simulink model "TL1_cs"  (R2019a)
settings: Solver=FixedStepDiscrete  StartTime=0.0  StopTime=40  FixedStep=1/300  RelTol=1e-3
PreLoadFcn:
  | mbxruntime.callbacks.PreLoadFcn(bdroot);
  | check_NUTS_defined
  | model_closed = 0;
  | assignin('base',['model_closed_' bdroot],false);
PostLoadFcn:
  | mbxruntime.callbacks.PostLoadFcn(bdroot);
InitFcn:
  | mbxruntime.callbacks.InitFcn(bdroot);
StartFcn:
  | mbxruntime.callbacks.StartFcn(bdroot);
StopFcn:
  | mbxruntime.callbacks.StopFcn(bdroot);;
  | 
model workspace: external: MAT-File .\TL1_cs_hws.mat (data not in the file)
undefined symbols (not defined in the file): AngularVelocity, Clock_, Data, Data_SL_Info, DiscIntNeverNeededParam, Encoding, Encoding_SL_Info, Header, Height, InitImageOutputDir, LinearAcceleration, mbxruntime, Orientation, Pose, Poses, Poses_SL_Info, Position, Step, tabledata, Twist, Width
libraries: robotlib x24, simulink_extras x16, PreScanSimulinkLibrary x4, dspindex x4, robotcorelib x2, visionconversions x2, visionsinks x2, sharedtransform x1
(part 2 of 4)

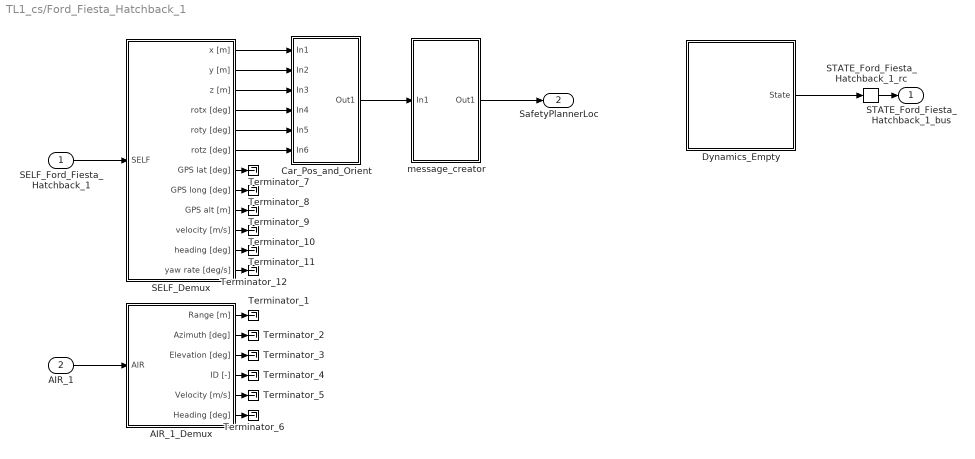
== system TL1_cs/Ford_Fiesta_Hatchback_1 ==
  SELF_Ford_Fiesta_Hatchback_1 : Inport  Tag=inport/SelfPort  OutDataTypeStr=Bus: PRESCAN_SELFSENSORDATA  PortDimensions=1  SampleTime=1/300  BusOutputAsStruct=on
  AIR_1 : Inport  Tag=inport/AIR  Port=2  OutDataTypeStr=Bus: PRESCAN_AIRSENSORMESSAGE  PortDimensions=1  SampleTime=1/300  BusOutputAsStruct=on
  AIR_1_Demux : Subsystem  Tag=demux/AIR  mask(PreScan Demux Block: AIR){DetectionType=BBox, detectableObjects=1}
      mask prompts: DetectionType "Detection Type"; detectableObjects "Max. detectable objects"
      mask help:
      | The Actor Information Receiver sensor provides a fast, simple and generic detection solution which is not tied up to a specific technology and can be used for scenarios in which a simple sensor is needed.
      |
      | For more information, please click Help.
      mask init:
      | switch DetectionType
      |     case 1
      |         DetectionTypeStr = 'Center';
      |     case 2
      |         DetectionTypeStr = 'BBox';
      |     case 3
      |         DetectionTypeStr = 'CoG';
      |     otherwise
      |         DetectionTypeStr = 'Unknown';
      | end
      settings: DeleteFcn=PreScanBlockDeleteFcn;
      mask Help: eval('openHelp(413)')
      mask TypeOptions DetectionType: Center | BBox | CoG
      mask Display:
      | disp(char('Det. type:         ',['{\it',DetectionTypeStr,'}']),'texmode','on')
      | port_label('output',1,'Range [m]')
      | port_label('output',2,'{\theta} [deg]','texmode','on')
      | port_label('output',3,'{\phi} [deg]','texmode','on')
      | port_label('output',4,'ID [-]','texmode','on')
      | port_label('output',5,'Velocity [m/s]','texmode','on')
      | port_label('output',6,'Heading [deg]','texmode','on')
  Car_Pos_and_Orient : Subsystem
  Dynamics_Empty : Subsystem  Tag=Dynamics_Empty
      mask Help: eval('openHelp(202)')
      mask Display: port_label('output', 1, 'State');text(0,0,' Empty\n')
  SELF_Demux : Subsystem  Tag=demux/SelfPort  mask(PreScan Demux Block:){}
      mask help:
      | The SELF port shows (state) information of the actor itself. The outputs are position in the experiment's axis system and the GPS coordinates, and the object's absolute velocity and compass heading.
      |
      | For more information, please click Help.
      settings: DeleteFcn=PreScanBlockDeleteFcn;
      mask Help: eval('openHelp(462)')
      mask Display:
      | port_label('output',1,'x [m]')
      | port_label('output',2,'y [m]')
      | port_label('output',3,'z [m]','texmode','on')
      | port_label('output',4,'Rotx [deg]','texmode','on')
      | port_label('output',5,'Roty [deg]','texmode','on')
      | port_label('output',6,'Rotz [deg]','texmode','on')
      | port_label('output',7,'GPS lat [deg]','texmode','on')
      | port_label('output',8,'GPS long [deg]','texmode','on')
      | port_label('output',9,'GPS alt [m]','texmode','on')
      | port_label('output',10,'Velocity [m/s]')
      | port_label('output',11,'Heading [deg]')
      | port_label('output',12,'Yaw rate [deg/s]')
  STATE_Ford_Fiesta_Hatchback_1_rc : RateTransition  Tag=mux_rc/StatePort  OutPortSampleTimeOpt=Inherit
  Terminator_{1..12} (12 alike) : Terminator
  message_creator : Subsystem
  STATE_Ford_Fiesta_Hatchback_1_bus : Outport  Tag=outport/StatePort  OutDataTypeStr=Bus: PRESCAN_STATEACTUATORDATA  PortDimensions=1  SampleTime=1/300
  SafetyPlannerLoc : Outport  Port=2
  wires:
  Car_Pos_and_Orient/1(Out1) -> message_creator/1(In1)
  message_creator/1(Out1) -> SafetyPlannerLoc/1
  SELF_Demux/1(x [m]) -> Car_Pos_and_Orient/1(In1)
  SELF_Demux/2(y [m]) -> Car_Pos_and_Orient/2(In2)
  SELF_Demux/3(z [m]) -> Car_Pos_and_Orient/3(In3)
  SELF_Demux/4(rotx [deg]) -> Car_Pos_and_Orient/4(In4)
  SELF_Demux/5(roty [deg]) -> Car_Pos_and_Orient/5(In5)
  SELF_Demux/6(rotz [deg]) -> Car_Pos_and_Orient/6(In6)
  STATE_Ford_Fiesta_Hatchback_1_rc/1 -> STATE_Ford_Fiesta_Hatchback_1_bus/1
  SELF_Ford_Fiesta_Hatchback_1/1 -> SELF_Demux/1(SELF)
  AIR_1/1 -> AIR_1_Demux/1(AIR)
  Dynamics_Empty/1(State) -> STATE_Ford_Fiesta_Hatchback_1_rc/1
  AIR_1_Demux/1(Range [m]) -> Terminator_1/1
  AIR_1_Demux/2(Azimuth [deg]) -> Terminator_2/1
  AIR_1_Demux/3(Elevation [deg]) -> Terminator_3/1
  AIR_1_Demux/4(ID [-]) -> Terminator_4/1
  AIR_1_Demux/5(Velocity [m/s]) -> Terminator_5/1
  AIR_1_Demux/6(Heading [deg]) -> Terminator_6/1
  SELF_Demux/7(GPS lat [deg]) -> Terminator_7/1
  SELF_Demux/8(GPS long [deg]) -> Terminator_8/1
  SELF_Demux/9(GPS alt [m]) -> Terminator_9/1
  SELF_Demux/10(velocity [m/s]) -> Terminator_10/1
  SELF_Demux/11(heading [deg]) -> Terminator_11/1
  SELF_Demux/12(yaw rate [deg/s]) -> Terminator_12/1

== system TL1_cs/HumViewCamera ==
  Sensor : S-Function  FunctionName=sfun_Camera  Parameters=sensorID, dataWidth, dataHeight, channelsPerImage, numberOfImages, timestep  SFunctionDeploymentMode=off  EnableBusSupport=off  mask(PreScan Source Block: Camera Sensor){sensorID=14458, dataWidth=1080, dataHeight=5613, channelsPerImage=3, numberOfImages=1, timestep=1/60}
      mask prompts: sensorID "Sensor ID"; dataWidth "Data width"; dataHeight "Data Height"; channelsPerImage "Channels per image"; numberOfImages "Number of images"; timestep "MATLAB timestep:"
      mask help: The Camera Sensor provides a color or monochrome image.
      mask Help: eval('openHelp(457)')
      mask Display: image(imread('CameraSensor.png'))
  HumViewCamera : Outport  Tag=outport/Camera/CameraSensor  OutDataTypeStr=uint8  SampleTime=1/60
  wires:
  Sensor/1 -> HumViewCamera/1

== system TL1_cs/PointCloudSensor_1 ==
  Sensor : S-Function  FunctionName=sfun_PCS  Parameters=sensorID, dataWidth, dataHeight, numChannels, dataType, timestep  SFunctionDeploymentMode=off  EnableBusSupport=off  mask(PreScan Source Block: Point Cloud Sensor){sensorID=9052, dataWidth=16, dataHeight=900, numChannels=4, dataType=0, timestep=1/20}
      mask prompts: sensorID "Sensor ID"; dataWidth "Data Width"; dataHeight "Data Height"; numChannels "Channel Count"; dataType "Data Type"; timestep "MATLAB timestep:"
      mask help: The Point Cloud Sensor provides XYZ positions relative to the sensor
      mask Help: eval('openHelp(6400)')
      mask Display: image(imread('PointCloudSensorSL.png'))
  PointCloudSensor_1 : Outport  Tag=outport/PointCloudInport  OutDataTypeStr=single  SampleTime=1/20
  wires:
  Sensor/1 -> PointCloudSensor_1/1

== system TL1_cs/PointCloudSensor_2 ==
  Sensor : S-Function  FunctionName=sfun_PCS  Parameters=sensorID, dataWidth, dataHeight, numChannels, dataType, timestep  SFunctionDeploymentMode=off  EnableBusSupport=off  mask(PreScan Source Block: Point Cloud Sensor){sensorID=9053, dataWidth=16, dataHeight=900, numChannels=4, dataType=0, timestep=1/20}
      mask prompts: sensorID "Sensor ID"; dataWidth "Data Width"; dataHeight "Data Height"; numChannels "Channel Count"; dataType "Data Type"; timestep "MATLAB timestep:"
      mask help: The Point Cloud Sensor provides XYZ positions relative to the sensor
      mask Help: eval('openHelp(6400)')
      mask Display: image(imread('PointCloudSensorSL.png'))
  PointCloudSensor_2 : Outport  Tag=outport/PointCloudInport  OutDataTypeStr=single  SampleTime=1/20
  wires:
  Sensor/1 -> PointCloudSensor_2/1

== system TL1_cs/PointCloudSensor_3 ==
  Sensor : S-Function  FunctionName=sfun_PCS  Parameters=sensorID, dataWidth, dataHeight, numChannels, dataType, timestep  SFunctionDeploymentMode=off  EnableBusSupport=off  mask(PreScan Source Block: Point Cloud Sensor){sensorID=9054, dataWidth=16, dataHeight=900, numChannels=4, dataType=0, timestep=1/20}
      mask prompts: sensorID "Sensor ID"; dataWidth "Data Width"; dataHeight "Data Height"; numChannels "Channel Count"; dataType "Data Type"; timestep "MATLAB timestep:"
      mask help: The Point Cloud Sensor provides XYZ positions relative to the sensor
      mask Help: eval('openHelp(6400)')
      mask Display: image(imread('PointCloudSensorSL.png'))
  PointCloudSensor_3 : Outport  Tag=outport/PointCloudInport  OutDataTypeStr=single  SampleTime=1/20
  wires:
  Sensor/1 -> PointCloudSensor_3/1

== system TL1_cs/PointCloudSensor_4 ==
  Sensor : S-Function  FunctionName=sfun_PCS  Parameters=sensorID, dataWidth, dataHeight, numChannels, dataType, timestep  SFunctionDeploymentMode=off  EnableBusSupport=off  mask(PreScan Source Block: Point Cloud Sensor){sensorID=9055, dataWidth=16, dataHeight=900, numChannels=4, dataType=0, timestep=1/20}
      mask prompts: sensorID "Sensor ID"; dataWidth "Data Width"; dataHeight "Data Height"; numChannels "Channel Count"; dataType "Data Type"; timestep "MATLAB timestep:"
      mask help: The Point Cloud Sensor provides XYZ positions relative to the sensor
      mask Help: eval('openHelp(6400)')
      mask Display: image(imread('PointCloudSensorSL.png'))
  PointCloudSensor_4 : Outport  Tag=outport/PointCloudInport  OutDataTypeStr=single  SampleTime=1/20
  wires:
  Sensor/1 -> PointCloudSensor_4/1

== system TL1_cs/PreScanTerminator ==
  Terminator : Terminator
  sfun_Terminator : S-Function  FunctionName=sfun_Terminator  Parameters=SampleTime  SFunctionDeploymentMode=off  EnableBusSupport=off  mask(Legacy Function){SFunctionSpec=void prescan_terminator_outputFcn(void ** work1, PRESCAN_TERMINATORDATA y1[1]), SampleTime=TimeStep, ShowSpec=on}
      mask prompts: SampleTime "Sample time (-1 for inherited):"; ShowSpec "Display function specification"
      mask help:
      | This block allows you to call the legacy functions specified by the following Legacy Code Tool definition:
      | def.SFunctionName = 'sfun_Terminator';
      | def.OutputFcnSpec = 'void prescan_terminator_outputFcn(void ** work1, PRESCAN_TERMINATORDATA y1[1])';
      | def.StartFcnSpec = 'void prescan_terminator_startFcn(void ** work1)';
      | def.TerminateFcnSpec = 'void prescan_terminator_terminateFcn(void ** work1)';
      | def.HeaderFiles = {'prescan_terminator_data.h'};
      | def.HostLibFiles = {'sensorinterfaced.lib'};
      | def.IncPaths = {'src', 'C:\prescandev\vislibrary\vis\..\pimp\include\sensors\InterfaceRTW'};
      | def.SrcPaths = {'src'};
      | def.LibPaths = {'C:\\prescandev\\vislibrary_build\lib'};
      | def.SampleTime = 'parameterized';
      | def.Options.language = 'C';
      mask Help: <p>This block was generated automatically by the Legacy Code Tool. For detailed help on this tool, call<a href="matlab:legacy_code('help')"> legacy_code('help')</a>.</p>
      mask Callback ShowSpec:
      | if strcmp(get_param(gcbh, 'ShowSpec'), 'on')
      |   set_param(gcbh, 'MaskDisplay', sprintf('fprintf(''%s'');', get_param(gcbh, 'SFunctionSpec')));
      | else
      |   set_param(gcbh, 'MaskDisplay', sprintf('fprintf(''%s'');', get_param(gcbh, 'FunctionName')));
      | end
      mask Display: fprintf('void prescan_terminator_outputFcn(void ** work1, PRESCAN_TERMINATORDATA y1[1])');
  wires:
  sfun_Terminator/1 -> Terminator/1

== system TL1_cs/SELF_BMW_X5_SUV_1 ==
  Sensor : S-Function  FunctionName=sfun_SelfSensor  Parameters=UniqueID, TimeStep  SFunctionDeploymentMode=off  EnableBusSupport=off  mask(PreScan Source Block: SELF){UniqueID=9040, TimeStep=1/300}
      mask prompts: UniqueID "Auto-Assigned: Unique ID"; TimeStep "Auto-Assigned: Upload Period [s]"
      mask help:
      | The SELF port shows (state) information of the actor itself. The outputs are position in the experiment's axis system and the GPS coordinates, and the object's absolute velocity and compass heading.
      |
      | For more information, please click Help.
      mask Help: eval('openHelp(462)')
      mask Display: image(imread('GPS.png'))
  SELF_BMW_X5_SUV_1 : Outport  Tag=outport/SelfPort  OutDataTypeStr=Bus: PRESCAN_SELFSENSORDATA  PortDimensions=1  SampleTime=1/300
  wires:
  Sensor/1 -> SELF_BMW_X5_SUV_1/1

== system TL1_cs/SELF_Ford_Fiesta_Hatchback_1 ==
  Sensor : S-Function  FunctionName=sfun_SelfSensor  Parameters=UniqueID, TimeStep  SFunctionDeploymentMode=off  EnableBusSupport=off  mask(PreScan Source Block: SELF){UniqueID=4876, TimeStep=1/300}
      mask prompts: UniqueID "Auto-Assigned: Unique ID"; TimeStep "Auto-Assigned: Upload Period [s]"
      mask help:
      | The SELF port shows (state) information of the actor itself. The outputs are position in the experiment's axis system and the GPS coordinates, and the object's absolute velocity and compass heading.
      |
      | For more information, please click Help.
      mask Help: eval('openHelp(462)')
      mask Display: image(imread('GPS.png'))
  SELF_Ford_Fiesta_Hatchback_1 : Outport  Tag=outport/SelfPort  OutDataTypeStr=Bus: PRESCAN_SELFSENSORDATA  PortDimensions=1  SampleTime=1/300
  wires:
  Sensor/1 -> SELF_Ford_Fiesta_Hatchback_1/1

== system TL1_cs/STATE_BMW_X5_SUV_1_bus ==
  STATE_BMW_X5_SUV_1_bus : Inport  Tag=inport/StatePort  OutDataTypeStr=Bus: PRESCAN_STATEACTUATORDATA  PortDimensions=1  SampleTime=1/300  BusOutputAsStruct=on
  Actuator : S-Function  FunctionName=sfun_StateActuator  Parameters=UniqueID, TimeStep  SFunctionDeploymentMode=off  EnableBusSupport=off  mask(PreScan Sink Block: State){UniqueID=9040, TimeStep=1/300}
      mask prompts: UniqueID "Auto-Assigned: Unique ID"; TimeStep "Auto-Assigned: Upload Period [s]"
      mask help:
      | The Actor State contains a vector signal of size (9x1), containing the following signals:
      |
      | -  Position    	(x,y,z)             	[m]
      | -  Velocity    	(vx,vy,vz)         	[m/s]
      | -  Angles       	(Roll, Pitch, Yaw)	[rad]
      |
      | The Actor state is defined in the global axis system.
      | The state is superponed on the Initial position defined in the GUI.
      |
      | For more information, please click Help.
      mask Help: eval('openHelp(222)')
      mask Display: image(imread('State.png'))
  wires:
  STATE_BMW_X5_SUV_1_bus/1 -> Actuator/1

== system TL1_cs/STATE_Ford_Fiesta_Hatchback_1_bus ==
  STATE_Ford_Fiesta_Hatchback_1_bus : Inport  Tag=inport/StatePort  OutDataTypeStr=Bus: PRESCAN_STATEACTUATORDATA  PortDimensions=1  SampleTime=1/300  BusOutputAsStruct=on
  Actuator : S-Function  FunctionName=sfun_StateActuator  Parameters=UniqueID, TimeStep  SFunctionDeploymentMode=off  EnableBusSupport=off  mask(PreScan Sink Block: State){UniqueID=4876, TimeStep=1/300}
      mask prompts: UniqueID "Auto-Assigned: Unique ID"; TimeStep "Auto-Assigned: Upload Period [s]"
      mask help:
      | The Actor State contains a vector signal of size (9x1), containing the following signals:
      |
      | -  Position    	(x,y,z)             	[m]
      | -  Velocity    	(vx,vy,vz)         	[m/s]
      | -  Angles       	(Roll, Pitch, Yaw)	[rad]
      |
      | The Actor state is defined in the global axis system.
      | The state is superponed on the Initial position defined in the GUI.
      |
      | For more information, please click Help.
      mask Help: eval('openHelp(222)')
      mask Display: image(imread('State.png'))
  wires:
  STATE_Ford_Fiesta_Hatchback_1_bus/1 -> Actuator/1

== system TL1_cs/Synchronizer ==
  Bus Selector1 : BusSelector  OutputSignals=FederateStopped
  Stop Simulation : Stop
  sfun_Synchronizer : S-Function  FunctionName=sfun_Synchronizer  Parameters=SampleTime  SFunctionDeploymentMode=off  EnableBusSupport=off  mask(Legacy Function){SFunctionSpec=void prescan_synchronizer_outputFcn(void ** work1, PRESCAN_SYNCHRONIZEDATA y1[1]), SampleTime=TimeStep, ShowSpec=on}
      mask prompts: SampleTime "Sample time (-1 for inherited):"; ShowSpec "Display function specification"
      mask help:
      | This block allows you to call the legacy functions specified by the following Legacy Code Tool definition:
      | def.SFunctionName = 'sfun_Synchronizer';
      | def.OutputFcnSpec = 'void prescan_synchronizer_outputFcn(void ** work1, PRESCAN_SYNCHRONIZEDATA y1[1])';
      | def.StartFcnSpec = 'void prescan_synchronizer_startFcn(void ** work1)';
      | def.TerminateFcnSpec = 'void prescan_synchronizer_terminateFcn(void ** work1)';
      | def.HeaderFiles = {'prescan_synchronizer_data.h'};
      | def.HostLibFiles = {'sensorinterfaced.lib'};
      | def.IncPaths = {'src', 'C:\prescandev\vislibrary\vis\..\pimp\include\sensors\InterfaceRTW'};
      | def.SrcPaths = {'src'};
      | def.LibPaths = {'C:\\prescandev\\vislibrary_build\lib'};
      | def.SampleTime = 'parameterized';
      | def.Options.language = 'C';
      mask Help: <p>This block was generated automatically by the Legacy Code Tool. For detailed help on this tool, call<a href="matlab:legacy_code('help')"> legacy_code('help')</a>.</p>
      mask Callback ShowSpec:
      | if strcmp(get_param(gcbh, 'ShowSpec'), 'on')
      |   set_param(gcbh, 'MaskDisplay', sprintf('fprintf(''%s'');', get_param(gcbh, 'SFunctionSpec')));
      | else
      |   set_param(gcbh, 'MaskDisplay', sprintf('fprintf(''%s'');', get_param(gcbh, 'FunctionName')));
      | end
      mask Display: fprintf('void prescan_synchronizer_outputFcn(void ** work1, PRESCAN_SYNCHRONIZEDATA y1[1])');
  wires:
  Bus Selector1/1 -> Stop Simulation/1  "<FederateStopped>"
  sfun_Synchronizer/1 -> Bus Selector1/1

== system TL1_cs/TrafficLightRoadSideNL_1 ==
  Constant : Constant
  Ground_1 : Ground
  Ground_2 : Ground
  VISUCasingLights_Mux : Subsystem  Tag=mux/VisuCasingLights  mask(PreScan User Interface: VisuTrafficLight){}
      mask help:
      | The VisuTrafficLight block provides a way to animate traffic lights: switch on and off individual lights.
      |
      | For more information, please click Help.
      mask Help: eval('openHelp(731)')
  VISUCasingLights_TrafficLightRoadSideNL_1 : Outport  Tag=outport/VisuCasingLights  SampleTime=1/300
  wires:
  VISUCasingLights_Mux/1(VISUCasingLights_TrafficLightRoadSideNL_1) -> VISUCasingLights_TrafficLightRoadSideNL_1/1
  Ground_1/1 -> VISUCasingLights_Mux/1(Green [-])
  Ground_2/1 -> VISUCasingLights_Mux/2(Orange [-])
  Constant/1 -> VISUCasingLights_Mux/3(Red [-])

== system TL1_cs/VISUCasingLights_TrafficLightRoadSideNL_1 ==
  VISUCasingLights_TrafficLightRoadSideNL_1 : Inport  Tag=inport/VisuCasingLights  SampleTime=1/300  BusOutputAsStruct=on
  Actuator : Subsystem  mask(PreScan Sink Block: VisuTrafficLight){UniqueID=20538, ColorsObjectQuery=, Colors=[]}
      mask prompts: UniqueID "Parent Unique Identifier"; ColorsObjectQuery "Query for Color Object"; Colors "Matrix of colors"
      mask help:
      | The VisuTrafficLight block provides a way to animate traffic lights: switch on and off individual lights.
      |
      | For more information, please click Help.
      mask Help: eval('openHelp(731)')
      mask Display: image(imread('TrafficLightCasing.png'))
  wires:
  VISUCasingLights_TrafficLightRoadSideNL_1/1 -> Actuator/1(VISUCasingLights_TrafficLightRoadSideNL_1)

== system TL1_cs/camera ==
  Sensor : S-Function  FunctionName=sfun_Camera  Parameters=sensorID, dataWidth, dataHeight, channelsPerImage, numberOfImages, timestep  SFunctionDeploymentMode=off  EnableBusSupport=off  mask(PreScan Source Block: Camera Sensor){sensorID=9056, dataWidth=720, dataHeight=2880, channelsPerImage=3, numberOfImages=1, timestep=1/20}
      mask prompts: sensorID "Sensor ID"; dataWidth "Data width"; dataHeight "Data Height"; channelsPerImage "Channels per image"; numberOfImages "Number of images"; timestep "MATLAB timestep:"
      mask help: The Camera Sensor provides a color or monochrome image.
      mask Help: eval('openHelp(457)')
      mask Display: image(imread('CameraSensor.png'))
  camera : Outport  Tag=outport/Camera/CameraSensor  OutDataTypeStr=uint8  SampleTime=1/20
  wires:
  Sensor/1 -> camera/1

== system TL1_cs/pose_otheCar ==
  In1 : Inport
  Enable : EnablePort
  Add5 : Sum
  Assignment : Assignment  OutputInitialize=Specify size for each dimension in table  DiagnosticForDimensions=Warning  IndexOptions=Starting index (dialog)  Indices=1  OutputSizes=1
  Assignment2 : Assignment  OutputInitialize=Specify size for each dimension in table  DiagnosticForDimensions=Warning  IndexOptions=Starting index (dialog)  Indices=1  OutputSizes=1000
  Blank Message1 : robotlib/Blank Message  messageClass=Message  entityType=geometry_msgs/PoseArray  messageType=geometry_msgs/PoseArray  SampleTime=inf
      settings: SourceProductBaseCode=RO
  Bus Assignment3 : BusAssignment  AssignedSignals=Header.Seq,Header.FrameId,Header.FrameId_SL_Info.CurrentLength,Poses,Poses_SL_Info.CurrentLength
  Bus Selector : BusSelector  OutputSignals=Poses
  Bus Selector2 : BusSelector  OutputSignals=Header.FrameId
  Constant24 : Constant  OutDataTypeStr=uint32
  Constant25 : Constant  Value=uint8(['map'])
  Memory2 : Memory  InheritSampleTime=on
  Publish2 : robotlib/Publish  topicSource=Specify your own  topic=/pose_otherCar  messageType=geometry_msgs/PoseArray  messageQueueLength=1
      settings: SourceProductBaseCode=RO
  Width : Width  DataType=uint32
  Width5 : Width  DataType=uint32
  wires:
  Constant24/1 -> Add5/2
  Memory2/1 -> Add5/1
  Add5/1 -> Bus Assignment3/2, Memory2/1
  Width5/1 -> Bus Assignment3/4
  Assignment/1 -> Bus Assignment3/5, Width/1
  Width/1 -> Bus Assignment3/6
  Bus Selector/1 -> Assignment/1  "<Poses>"
  In1/1 -> Assignment/2
  Bus Assignment3/1 -> Publish2/1
  Constant25/1 -> Assignment2/2
  Assignment2/1 -> Bus Assignment3/3, Width5/1
  Bus Selector2/1 -> Assignment2/1  "<FrameId>"
  Blank Message1/1 -> Bus Selector/1, Bus Selector2/1, Bus Assignment3/1

== system TL1_cs/tl_camera ==
  Sensor : S-Function  FunctionName=sfun_Camera  Parameters=sensorID, dataWidth, dataHeight, channelsPerImage, numberOfImages, timestep  SFunctionDeploymentMode=off  EnableBusSupport=off  mask(PreScan Source Block: Camera Sensor){sensorID=12017, dataWidth=720, dataHeight=2880, channelsPerImage=3, numberOfImages=1, timestep=1/20}
      mask prompts: sensorID "Sensor ID"; dataWidth "Data width"; dataHeight "Data Height"; channelsPerImage "Channels per image"; numberOfImages "Number of images"; timestep "MATLAB timestep:"
      mask help: The Camera Sensor provides a color or monochrome image.
      mask Help: eval('openHelp(457)')
      mask Display: image(imread('CameraSensor.png'))
  tl_camera : Outport  Tag=outport/Camera/CameraSensor  OutDataTypeStr=uint8  SampleTime=1/20
  wires:
  Sensor/1 -> tl_camera/1

== system TL1_cs/BMW_X5_SUV_1/Car_Pose ==
  In1 : Inport
  In2 : Inport  Port=2
  In3 : Inport  Port=3
  In4 : Inport  Port=4
  In5 : Inport  Port=5
  In6 : Inport  Port=6
  Coordinate Transformation Conversion : robotcorelib/Coordinate Transformation Conversion  InputRepresentation=Euler Angles  InputEulerSequence=XYZ  ShowTrVecInputPort=on  OutputRepresentation=Quaternion  OutputEulerSequence=ZYX  ShowTrVecOutputPort=on  SimulateUsing=Interpreted execution
      settings: SourceProductBaseCode=RO
  Data Type Conversion : DataTypeConversion
  Data Type Conversion1 : DataTypeConversion
  Data Type Conversion2 : DataTypeConversion
  Degrees to Radians1 : simulink_extras/Transformations/Degrees to Radians
  Degrees to Radians2 : simulink_extras/Transformations/Degrees to Radians
  Degrees to Radians5 : simulink_extras/Transformations/Degrees to Radians
  Mux : Mux
  Vector Concatenate2 : Concatenate  NumInputs=3
  Out1 : Outport
  wires:
  Mux/1 -> Out1/1
  Coordinate Transformation Conversion/1 -> Mux/4
  Data Type Conversion2/1 -> Mux/3
  Data Type Conversion1/1 -> Mux/2
  Data Type Conversion/1 -> Mux/1
  In6/1 -> Degrees to Radians2/1
  In5/1 -> Degrees to Radians1/1
  In4/1 -> Degrees to Radians5/1
  In3/1 -> Data Type Conversion2/1
  In2/1 -> Data Type Conversion1/1
  In1/1 -> Data Type Conversion/1
  Degrees to Radians2/1 -> Vector Concatenate2/3
  Vector Concatenate2/1 -> Coordinate Transformation Conversion/1
  Degrees to Radians5/1 -> Vector Concatenate2/1
  Degrees to Radians1/1 -> Vector Concatenate2/2

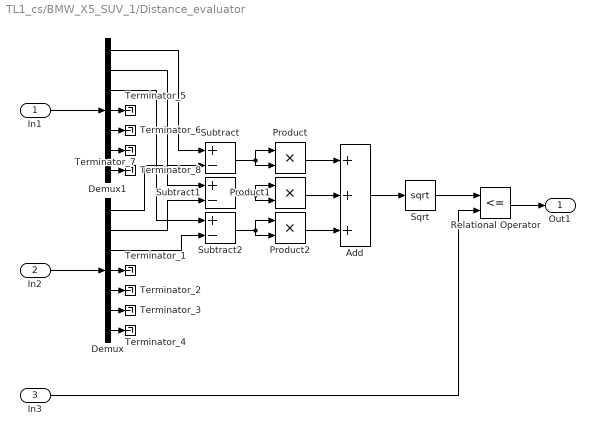
== system TL1_cs/BMW_X5_SUV_1/Distance_evaluator ==
  In1 : Inport
  In2 : Inport  Port=2
  In3 : Inport  Port=3
  Add : Sum  Inputs=3
  Demux : Demux  Outputs=7
  Demux1 : Demux  Outputs=7
  Product : Product
  Product1 : Product
  Product2 : Product
  Relational Operator : RelationalOperator  Operator=<=  OutDataTypeStr=boolean  RndMeth=Simplest
  Sqrt : Sqrt  SaturateOnIntegerOverflow=on
  Subtract : Sum  Inputs=+-
  Subtract1 : Sum  Inputs=+-
  Subtract2 : Sum  Inputs=+-
  Terminator_{1..8} (8 alike) : Terminator
  Out1 : Outport
  wires:
  Demux1/7 -> Terminator_8/1
  Demux1/6 -> Terminator_7/1
  Demux1/5 -> Terminator_6/1
  Demux1/4 -> Terminator_5/1
  Demux/7 -> Terminator_4/1
  Demux/6 -> Terminator_3/1
  Demux/5 -> Terminator_2/1
  Demux/4 -> Terminator_1/1
  In3/1 -> Relational Operator/2
  Sqrt/1 -> Relational Operator/1
  Add/1 -> Sqrt/1
  Product2/1 -> Add/3
  Product1/1 -> Add/2
  Product/1 -> Add/1
  Subtract2/1 -> Product2/2, Product2/1
  Subtract1/1 -> Product1/2, Product1/1
  Subtract/1 -> Product/2, Product/1
  Demux/3 -> Subtract2/2
  Demux/2 -> Subtract1/2
  Demux/1 -> Subtract/2
  Demux1/3 -> Subtract2/1
  Demux1/2 -> Subtract1/1
  Demux1/1 -> Subtract/1
  In2/1 -> Demux/1
  In1/1 -> Demux1/1
  Relational Operator/1 -> Out1/1

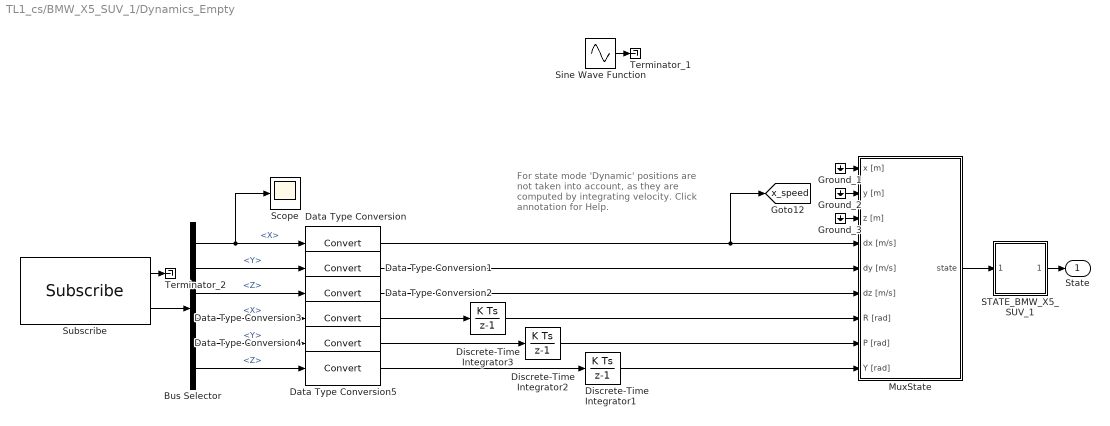
== system TL1_cs/BMW_X5_SUV_1/Dynamics_Empty ==
  note: For state mode 'Dynamic' positions
      | are not taken into account, as they
      | are computed by integrating velocity.
      | Click annotation for Help.
  Bus Selector : BusSelector  OutputSignals=Twist.Linear.X,Twist.Linear.Y,Twist.Linear.Z,Twist.Angular.X,Twist.Angular.Y,Twist.Angular.Z
  Data Type Conversion{,1..5} (6 alike) : DataTypeConversion
  Discrete-Time Integrator1 : DiscreteIntegrator  SampleTime=-1  ICPrevOutput=DiscIntNeverNeededParam  ICPrevScaledInput=DiscIntNeverNeededParam
  Discrete-Time Integrator2 : DiscreteIntegrator  SampleTime=-1  ICPrevOutput=DiscIntNeverNeededParam  ICPrevScaledInput=DiscIntNeverNeededParam
  Discrete-Time Integrator3 : DiscreteIntegrator  SampleTime=-1  ICPrevOutput=DiscIntNeverNeededParam  ICPrevScaledInput=DiscIntNeverNeededParam
  Ground_1 : Ground
  Ground_2 : Ground
  Ground_3 : Ground
  MuxState : Subsystem  Tag=mux/State  mask(Empty Dynamics State Block){positioningmode=off, TimeStep=1/300}
      mask prompts: positioningmode "Positioning Mode"; TimeStep "Auto Assigned: Time Step [s]"
      mask help:
      | Build the state of an actor based on user input.
      | The user can either use positioning mode or dynamics mode.
      | - When using positioning mode the position and orientation of the actor are set directly based on the input. Expected input is relative to the initial position and orientation of the actor. It's also possible to specify the velocity of the actor, though this input isn't used, only passed on.
      | - When using dynamics mode the position input is ignored. Expected input is velocity and orientation. The velocity is relative the current orientation of the actor, while orientation is relative to its initial orientation. The position of the actor is calculated based on the velocity and orientation given.
      settings: DeleteFcn=PreScanBlockDeleteFcn;
  STATE_BMW_X5_SUV_1 : Subsystem  Tag=mux/StatePort  Priority=0  LoadFcn=load PrescanStateActuatorData  mask(PreScan Sink Block: State){x0=0.12545, y0=2.1821, z0=0.69, Roll0=0, Pitch0=0, Yaw0=359.6217, TimeStep=1/300}
      mask prompts: x0 "Ini x-position VEHICLE wrt GLOBAL axis system [m]"; y0 "Ini y-position VEHICLE wrt GLOBAL axis system [m]"; z0 "Ini z-position VEHICLE wrt GLOBAL axis system [m]"; Roll0 "Ini roll-angle BODY wrt VEHICLE axis system [deg]"; Pitch0 "Ini pitch-angle BODY wrt VEHICLE axis system [deg]"; Yaw0 "Ini yaw-angle VEHICLE wrt GLOBAL axis system [deg]"; TimeStep "Auto-Assigned: Upload Period [s]"
      mask help:
      | The Actor State contains a vector signal of size (9x1), containing the following signals:
      |
      | -  Position                  (x,y,z)                                     [m]
      | -  Velocity                  (vx,vy,vz)                               [m/s]
      | -  Angles                    (Roll, Pitch, Yaw)                   [rad]
      |
      | The Actor state is defined in the global axis system.
      | The state is superponed on the Initial position defined in the GUI.
      |
      | For more information, please click Help.
      settings: DeleteFcn=PreScanBlockDeleteFcn;
      mask Help: eval('openHelp(222)')
      mask Display: image(imread('State.png'))
  Scope : Scope
  Sine Wave Function : Sin  Amplitude=0.1  SampleTime=0
  Subscribe : robotlib/Subscribe  topicSource=Select from ROS network  topic=/TwistS  messageType=geometry_msgs/TwistStamped  sampleTime=-1  messageQueueLength=1
      settings: SourceProductBaseCode=RO
  Terminator_1 : Terminator
  Terminator_2 : Terminator
  State : Outport  Tag=outport/StateOutport  SampleTime=1/300
  tag scope: x_speed=global
  wires:
  Bus Selector/1 -> Scope/1, Data Type Conversion/1  "<X>"
  Data Type Conversion/1 -> [x_speed], MuxState/4(dx [m/s])
  Bus Selector/2 -> Data Type Conversion1/1  "<Y>"
  Bus Selector/3 -> Data Type Conversion2/1  "<Z>"
  Bus Selector/4 -> Data Type Conversion3/1  "<X>"
  Data Type Conversion3/1 -> Discrete-Time Integrator3/1
  Bus Selector/5 -> Data Type Conversion4/1  "<Y>"
  Data Type Conversion4/1 -> Discrete-Time Integrator2/1
  Bus Selector/6 -> Data Type Conversion5/1  "<Z>"
  Data Type Conversion5/1 -> Discrete-Time Integrator1/1
  Subscribe/2 -> Bus Selector/1
  Data Type Conversion1/1 -> MuxState/5(dy [m/s])
  Data Type Conversion2/1 -> MuxState/6(dz [m/s])
  Discrete-Time Integrator3/1 -> MuxState/7(R [rad])
  Discrete-Time Integrator2/1 -> MuxState/8(P [rad])
  Discrete-Time Integrator1/1 -> MuxState/9(Y [rad])
  MuxState/1(state) -> STATE_BMW_X5_SUV_1/1(State)
  STATE_BMW_X5_SUV_1/1(StateBus) -> State/1
  Ground_1/1 -> MuxState/1(x [m])
  Ground_2/1 -> MuxState/2(y [m])
  Ground_3/1 -> MuxState/3(z [m])
  Sine Wave Function/1 -> Terminator_1/1
  Subscribe/1 -> Terminator_2/1

== system TL1_cs/BMW_X5_SUV_1/Frequency evaluator ==
  In1 : Inport
  Add : Sum  Inputs=+-
  Clock2 : Clock
  Constant : Constant
  Divide : Product  Inputs=*/
  Memory : Memory
  Relational Operator : RelationalOperator  OutDataTypeStr=boolean  RndMeth=Simplest
  Switch : Switch  Criteria=u2 > Threshold
  Out1 : Outport
  wires:
  Divide/1 -> Relational Operator/2
  Constant/1 -> Divide/1
  In1/1 -> Divide/2
  Clock2/1 -> Switch/1, Add/1
  Relational Operator/1 -> Out1/1, Switch/2
  Add/1 -> Relational Operator/1
  Switch/1 -> Memory/1
  Memory/1 -> Add/2, Switch/3

== system TL1_cs/BMW_X5_SUV_1/Frequency evaluator1 ==
  In1 : Inport
  Add : Sum  Inputs=+-
  Clock2 : Clock
  Constant : Constant
  Divide : Product  Inputs=*/
  Memory : Memory
  Relational Operator : RelationalOperator  OutDataTypeStr=boolean  RndMeth=Simplest
  Switch : Switch  Criteria=u2 > Threshold
  Out1 : Outport
  wires:
  Divide/1 -> Relational Operator/2
  Constant/1 -> Divide/1
  In1/1 -> Divide/2
  Clock2/1 -> Switch/1, Add/1
  Relational Operator/1 -> Out1/1, Switch/2
  Add/1 -> Relational Operator/1
  Switch/1 -> Memory/1
  Memory/1 -> Add/2, Switch/3

== system TL1_cs/BMW_X5_SUV_1/Frequency evaluator2 ==
  In1 : Inport
  Add : Sum  Inputs=+-
  Clock2 : Clock
  Constant : Constant
  Divide : Product  Inputs=*/
  Memory : Memory
  Relational Operator : RelationalOperator  OutDataTypeStr=boolean  RndMeth=Simplest
  Switch : Switch  Criteria=u2 > Threshold
  Out1 : Outport
  wires:
  Divide/1 -> Relational Operator/2
  Constant/1 -> Divide/1
  In1/1 -> Divide/2
  Clock2/1 -> Switch/1, Add/1
  Relational Operator/1 -> Out1/1, Switch/2
  Add/1 -> Relational Operator/1
  Switch/1 -> Memory/1
  Memory/1 -> Add/2, Switch/3

== system TL1_cs/BMW_X5_SUV_1/Frequency evaluator3 ==
  In1 : Inport
  Add : Sum  Inputs=+-
  Clock2 : Clock
  Constant : Constant
  Divide : Product  Inputs=*/
  Memory : Memory
  Relational Operator : RelationalOperator  OutDataTypeStr=boolean  RndMeth=Simplest
  Switch : Switch  Criteria=u2 > Threshold
  Out1 : Outport
  wires:
  Divide/1 -> Relational Operator/2
  Constant/1 -> Divide/1
  In1/1 -> Divide/2
  Clock2/1 -> Switch/1, Add/1
  Relational Operator/1 -> Out1/1, Switch/2
  Add/1 -> Relational Operator/1
  Switch/1 -> Memory/1
  Memory/1 -> Add/2, Switch/3

== system TL1_cs/BMW_X5_SUV_1/Frequency evaluator4 ==
  In1 : Inport
  Add : Sum  Inputs=+-
  Clock2 : Clock
  Constant : Constant
  Divide : Product  Inputs=*/
  Memory : Memory
  Relational Operator : RelationalOperator  OutDataTypeStr=boolean  RndMeth=Simplest
  Switch : Switch  Criteria=u2 > Threshold
  Out1 : Outport
  wires:
  Divide/1 -> Relational Operator/2
  Constant/1 -> Divide/1
  In1/1 -> Divide/2
  Clock2/1 -> Switch/1, Add/1
  Relational Operator/1 -> Out1/1, Switch/2
  Add/1 -> Relational Operator/1
  Switch/1 -> Memory/1
  Memory/1 -> Add/2, Switch/3

== system TL1_cs/BMW_X5_SUV_1/Frequency evaluator5 ==
  In1 : Inport
  Add : Sum  Inputs=+-
  Clock2 : Clock
  Constant : Constant
  Divide : Product  Inputs=*/
  Memory : Memory
  Relational Operator : RelationalOperator  OutDataTypeStr=boolean  RndMeth=Simplest
  Switch : Switch  Criteria=u2 > Threshold
  Out1 : Outport
  wires:
  Divide/1 -> Relational Operator/2
  Constant/1 -> Divide/1
  In1/1 -> Divide/2
  Clock2/1 -> Switch/1, Add/1
  Relational Operator/1 -> Out1/1, Switch/2
  Add/1 -> Relational Operator/1
  Switch/1 -> Memory/1
  Memory/1 -> Add/2, Switch/3

== system TL1_cs/BMW_X5_SUV_1/Frequency evaluator6 ==
  In1 : Inport
  Add : Sum  Inputs=+-
  Clock2 : Clock
  Constant : Constant
  Divide : Product  Inputs=*/
  Memory : Memory
  Relational Operator : RelationalOperator  OutDataTypeStr=boolean  RndMeth=Simplest
  Switch : Switch  Criteria=u2 > Threshold
  Out1 : Outport
  wires:
  Memory/1 -> Switch/3, Add/2
  Switch/1 -> Memory/1
  Add/1 -> Relational Operator/1
  Relational Operator/1 -> Switch/2, Out1/1
  Clock2/1 -> Add/1, Switch/1
  In1/1 -> Divide/2
  Constant/1 -> Divide/1
  Divide/1 -> Relational Operator/2

== system TL1_cs/BMW_X5_SUV_1/Frequency evaluator7 ==
  In1 : Inport
  Add : Sum  Inputs=+-
  Clock2 : Clock
  Constant : Constant
  Divide : Product  Inputs=*/
  Memory : Memory
  Relational Operator : RelationalOperator  OutDataTypeStr=boolean  RndMeth=Simplest
  Switch : Switch  Criteria=u2 > Threshold
  Out1 : Outport
  wires:
  Memory/1 -> Switch/3, Add/2
  Switch/1 -> Memory/1
  Add/1 -> Relational Operator/1
  Relational Operator/1 -> Switch/2, Out1/1
  Clock2/1 -> Add/1, Switch/1
  In1/1 -> Divide/2
  Constant/1 -> Divide/1
  Divide/1 -> Relational Operator/2

== system TL1_cs/BMW_X5_SUV_1/HumViewCamera_CM_Demux ==
  In1 : Inport
  Selector : Selector  NumberOfDimensions=2  InputPortWidth=3  IndexOptions=Index vector (dialog),Index vector (dialog)  Indices=-1,1:hres  OutputSizes=1,1
  Selector1 : Selector  NumberOfDimensions=2  InputPortWidth=3  IndexOptions=Index vector (dialog),Index vector (dialog)  Indices=-1,hres+1:hres*2  OutputSizes=1,1
  Selector2 : Selector  NumberOfDimensions=2  InputPortWidth=3  IndexOptions=Index vector (dialog),Index vector (dialog)  Indices=-1,hres*2+1:hres*3  OutputSizes=1,1
  R : Outport
  G : Outport  Port=2
  B : Outport  Port=3
  wires:
  In1/1 -> Selector1/1, Selector/1, Selector2/1
  Selector/1 -> R/1
  Selector1/1 -> G/1
  Selector2/1 -> B/1

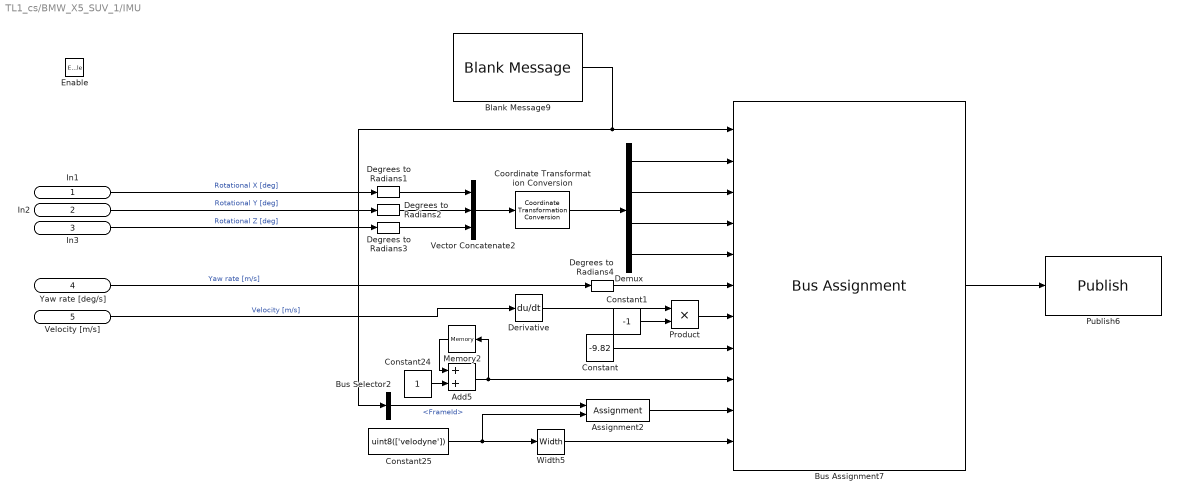
== system TL1_cs/BMW_X5_SUV_1/IMU ==
  In1 : Inport
  In2 : Inport  Port=2
  In3 : Inport  Port=3
  Yaw rate [deg/s] : Inport  Port=4
  Velocity [m/s] : Inport  Port=5
  Enable : EnablePort
  Add5 : Sum
  Assignment2 : Assignment  OutputInitialize=Specify size for each dimension in table  DiagnosticForDimensions=Warning  IndexOptions=Starting index (dialog)  Indices=1  OutputSizes=1000
  Blank Message9 : robotlib/Blank Message  messageClass=Message  entityType=sensor_msgs/Imu  messageType=sensor_msgs/Imu  SampleTime=inf
      settings: SourceProductBaseCode=RO
  Bus Assignment7 : BusAssignment  AssignedSignals=Orientation.W,Orientation.X,Orientation.Y,Orientation.Z,AngularVelocity.Z,LinearAcceleration.X,LinearAcceleration.Z,Header.Seq,Header.FrameId,Header.FrameId_SL_Info.CurrentLength
  Bus Selector2 : BusSelector  OutputSignals=Header.FrameId
  Constant : Constant  Value=-9.82
  Constant1 : Constant  Value=-1
  Constant24 : Constant  OutDataTypeStr=uint32
  Constant25 : Constant  Value=uint8(['velodyne'])
  Coordinate Transformation Conversion : robotcorelib/Coordinate Transformation Conversion  InputRepresentation=Euler Angles  InputEulerSequence=XYZ  ShowTrVecInputPort=on  OutputRepresentation=Quaternion  OutputEulerSequence=ZYX  ShowTrVecOutputPort=on  SimulateUsing=Interpreted execution
      settings: SourceProductBaseCode=RO
  Degrees to Radians{1..4} (4 alike) : simulink_extras/Transformations/Degrees to Radians
  Demux : Demux
  Derivative : Derivative
  Memory2 : Memory  InheritSampleTime=on
  Product : Product
  Publish6 : robotlib/Publish  topicSource=Select from ROS network  topic=/imu_raw  messageType=sensor_msgs/Imu  messageQueueLength=1
      settings: SourceProductBaseCode=RO
  Vector Concatenate2 : Concatenate  NumInputs=3
  Width5 : Width  DataType=uint32
  wires:
  Degrees to Radians1/1 -> Vector Concatenate2/1
  Constant24/1 -> Add5/2
  Constant25/1 -> Assignment2/2, Width5/1
  Bus Selector2/1 -> Assignment2/1  "<FrameId>"
  Blank Message9/1 -> Bus Selector2/1, Bus Assignment7/1
  Width5/1 -> Bus Assignment7/11
  Add5/1 -> Memory2/1, Bus Assignment7/9
  Bus Assignment7/1 -> Publish6/1
  Memory2/1 -> Add5/1
  Degrees to Radians4/1 -> Bus Assignment7/6
  Assignment2/1 -> Bus Assignment7/10
  Derivative/1 -> Product/1
  Degrees to Radians2/1 -> Vector Concatenate2/2
  Demux/2 -> Bus Assignment7/3
  Degrees to Radians3/1 -> Vector Concatenate2/3
  Vector Concatenate2/1 -> Coordinate Transformation Conversion/1
  Demux/3 -> Bus Assignment7/4
  Coordinate Transformation Conversion/1 -> Demux/1
  Demux/1 -> Bus Assignment7/2
  Demux/4 -> Bus Assignment7/5
  Yaw rate [deg/s]/1 -> Degrees to Radians4/1  "Yaw rate [m/s]"
  Velocity [m/s]/1 -> Derivative/1  "Velocity [m/s]"
  Constant/1 -> Bus Assignment7/8
  In1/1 -> Degrees to Radians1/1  "Rotational X [deg]"
  In2/1 -> Degrees to Radians2/1  "Rotational Y [deg]"
  In3/1 -> Degrees to Radians3/1  "Rotational Z [deg]"
  Constant1/1 -> Product/2
  Product/1 -> Bus Assignment7/7

== system TL1_cs/BMW_X5_SUV_1/PointCloudSensor_1_Angles_Demux ==
  In2 : Inport
  Selector : Selector  NumberOfDimensions=2  InputPortWidth=3  IndexOptions=Index vector (dialog),Index vector (dialog)  Indices=-1,offset+1:(offset+hres)  OutputSizes=1,1
  Selector1 : Selector  NumberOfDimensions=2  InputPortWidth=3  IndexOptions=Index vector (dialog),Index vector (dialog)  Indices=-1,(offset+hres+1):(offset+2*hres)  OutputSizes=1,1
  Theta : Outport
  Phi : Outport  Port=2
  wires:
  Selector1/1 -> Phi/1
  Selector/1 -> Theta/1
  In2/1 -> Selector/1, Selector1/1

== system TL1_cs/BMW_X5_SUV_1/PointCloudSensor_1_Intensity_Demux ==
  In1 : Inport
  Selector3 : Selector  NumberOfDimensions=2  InputPortWidth=3  IndexOptions=Index vector (dialog),Index vector (dialog)  Indices=-1,offset+1:(offset+hres)  OutputSizes=1,1
  Intensity : Outport
  wires:
  Selector3/1 -> Intensity/1
  In1/1 -> Selector3/1

== system TL1_cs/BMW_X5_SUV_1/PointCloudSensor_1_Range_Demux ==
  In1 : Inport
  Selector : Selector  NumberOfDimensions=2  InputPortWidth=3  IndexOptions=Index vector (dialog),Index vector (dialog)  Indices=-1,offset+1:(offset+hres)  OutputSizes=1,1
  Range : Outport
  wires:
  Selector/1 -> Range/1
  In1/1 -> Selector/1

== system TL1_cs/BMW_X5_SUV_1/PointCloudSensor_2_Angles_Demux ==
  In2 : Inport
  Selector : Selector  NumberOfDimensions=2  InputPortWidth=3  IndexOptions=Index vector (dialog),Index vector (dialog)  Indices=-1,offset+1:(offset+hres)  OutputSizes=1,1
  Selector1 : Selector  NumberOfDimensions=2  InputPortWidth=3  IndexOptions=Index vector (dialog),Index vector (dialog)  Indices=-1,(offset+hres+1):(offset+2*hres)  OutputSizes=1,1
  Theta : Outport
  Phi : Outport  Port=2
  wires:
  Selector1/1 -> Phi/1
  Selector/1 -> Theta/1
  In2/1 -> Selector/1, Selector1/1

== system TL1_cs/BMW_X5_SUV_1/PointCloudSensor_2_Intensity_Demux ==
  In1 : Inport
  Selector3 : Selector  NumberOfDimensions=2  InputPortWidth=3  IndexOptions=Index vector (dialog),Index vector (dialog)  Indices=-1,offset+1:(offset+hres)  OutputSizes=1,1
  Intensity : Outport
  wires:
  Selector3/1 -> Intensity/1
  In1/1 -> Selector3/1

== system TL1_cs/BMW_X5_SUV_1/PointCloudSensor_2_Range_Demux ==
  In1 : Inport
  Selector : Selector  NumberOfDimensions=2  InputPortWidth=3  IndexOptions=Index vector (dialog),Index vector (dialog)  Indices=-1,offset+1:(offset+hres)  OutputSizes=1,1
  Range : Outport
  wires:
  Selector/1 -> Range/1
  In1/1 -> Selector/1

== system TL1_cs/BMW_X5_SUV_1/PointCloudSensor_3_Angles_Demux ==
  In2 : Inport
  Selector : Selector  NumberOfDimensions=2  InputPortWidth=3  IndexOptions=Index vector (dialog),Index vector (dialog)  Indices=-1,offset+1:(offset+hres)  OutputSizes=1,1
  Selector1 : Selector  NumberOfDimensions=2  InputPortWidth=3  IndexOptions=Index vector (dialog),Index vector (dialog)  Indices=-1,(offset+hres+1):(offset+2*hres)  OutputSizes=1,1
  Theta : Outport
  Phi : Outport  Port=2
  wires:
  Selector1/1 -> Phi/1
  Selector/1 -> Theta/1
  In2/1 -> Selector/1, Selector1/1

== system TL1_cs/BMW_X5_SUV_1/PointCloudSensor_3_Intensity_Demux ==
  In1 : Inport
  Selector3 : Selector  NumberOfDimensions=2  InputPortWidth=3  IndexOptions=Index vector (dialog),Index vector (dialog)  Indices=-1,offset+1:(offset+hres)  OutputSizes=1,1
  Intensity : Outport
  wires:
  Selector3/1 -> Intensity/1
  In1/1 -> Selector3/1

== system TL1_cs/BMW_X5_SUV_1/PointCloudSensor_3_Range_Demux ==
  In1 : Inport
  Selector : Selector  NumberOfDimensions=2  InputPortWidth=3  IndexOptions=Index vector (dialog),Index vector (dialog)  Indices=-1,offset+1:(offset+hres)  OutputSizes=1,1
  Range : Outport
  wires:
  Selector/1 -> Range/1
  In1/1 -> Selector/1

== system TL1_cs/BMW_X5_SUV_1/PointCloudSensor_4_Angles_Demux ==
  In2 : Inport
  Selector : Selector  NumberOfDimensions=2  InputPortWidth=3  IndexOptions=Index vector (dialog),Index vector (dialog)  Indices=-1,offset+1:(offset+hres)  OutputSizes=1,1
  Selector1 : Selector  NumberOfDimensions=2  InputPortWidth=3  IndexOptions=Index vector (dialog),Index vector (dialog)  Indices=-1,(offset+hres+1):(offset+2*hres)  OutputSizes=1,1
  Theta : Outport
  Phi : Outport  Port=2
  wires:
  Selector1/1 -> Phi/1
  Selector/1 -> Theta/1
  In2/1 -> Selector/1, Selector1/1

== system TL1_cs/BMW_X5_SUV_1/PointCloudSensor_4_Intensity_Demux ==
  In1 : Inport
  Selector3 : Selector  NumberOfDimensions=2  InputPortWidth=3  IndexOptions=Index vector (dialog),Index vector (dialog)  Indices=-1,offset+1:(offset+hres)  OutputSizes=1,1
  Intensity : Outport
  wires:
  Selector3/1 -> Intensity/1
  In1/1 -> Selector3/1

== system TL1_cs/BMW_X5_SUV_1/PointCloudSensor_4_Range_Demux ==
  In1 : Inport
  Selector : Selector  NumberOfDimensions=2  InputPortWidth=3  IndexOptions=Index vector (dialog),Index vector (dialog)  Indices=-1,offset+1:(offset+hres)  OutputSizes=1,1
  Range : Outport
  wires:
  Selector/1 -> Range/1
  In1/1 -> Selector/1

== system TL1_cs/BMW_X5_SUV_1/SELF_Demux ==
  SELF : Inport  OutDataTypeStr=Bus: PRESCAN_SELFSENSORDATA
  Bus Selector : BusSelector  OutputSignals=PositionX,PositionY,PositionZ,OrientationRoll,OrientationPitch,OrientationYaw,Velocity,Yaw_rate,Lat,Long,Alt
  Demux2 : Demux  Outputs=3
  Gain : Gain  Gain=180/pi
  Gain1 : Gain  Gain=180/pi
  Vector Concatenate1 : Concatenate  NumInputs=3
  compas converter : Subsystem
  x [m] : Outport
  y [m] : Outport  Port=2
  z [m] : Outport  Port=3
  rotx [deg] : Outport  Port=4
  roty [deg] : Outport  Port=5
  rotz [deg] : Outport  Port=6
  GPS lat [deg] : Outport  Port=7
  GPS long [deg] : Outport  Port=8
  GPS alt [m] : Outport  Port=9
  velocity [m/s] : Outport  Port=10
  heading [deg] : Outport  Port=11
  yaw rate [deg/s] : Outport  Port=12
  wires:
  Bus Selector/11 -> GPS alt [m]/1  "<Alt>"
  Bus Selector/10 -> GPS long [deg]/1  "<Long>"
  Bus Selector/9 -> GPS lat [deg]/1  "<Lat>"
  Bus Selector/8 -> Gain1/1  "<Yaw_rate>"
  Bus Selector/7 -> velocity [m/s]/1  "<Velocity>"
  Bus Selector/6 -> compas converter/1(rotz [rad]), Vector Concatenate1/3  "<OrientationYaw>"
  Bus Selector/5 -> Vector Concatenate1/2  "<OrientationPitch>"
  Bus Selector/4 -> Vector Concatenate1/1  "<OrientationRoll>"
  Vector Concatenate1/1 -> Gain/1
  Bus Selector/3 -> z [m]/1  "<PositionZ>"
  Bus Selector/2 -> y [m]/1  "<PositionY>"
  Bus Selector/1 -> x [m]/1  "<PositionX>"
  SELF/1 -> Bus Selector/1
  Gain/1 -> Demux2/1
  Demux2/1 -> rotx [deg]/1
  Demux2/2 -> roty [deg]/1
  Demux2/3 -> rotz [deg]/1
  compas converter/1(heading [deg]) -> heading [deg]/1
  Gain1/1 -> yaw rate [deg/s]/1

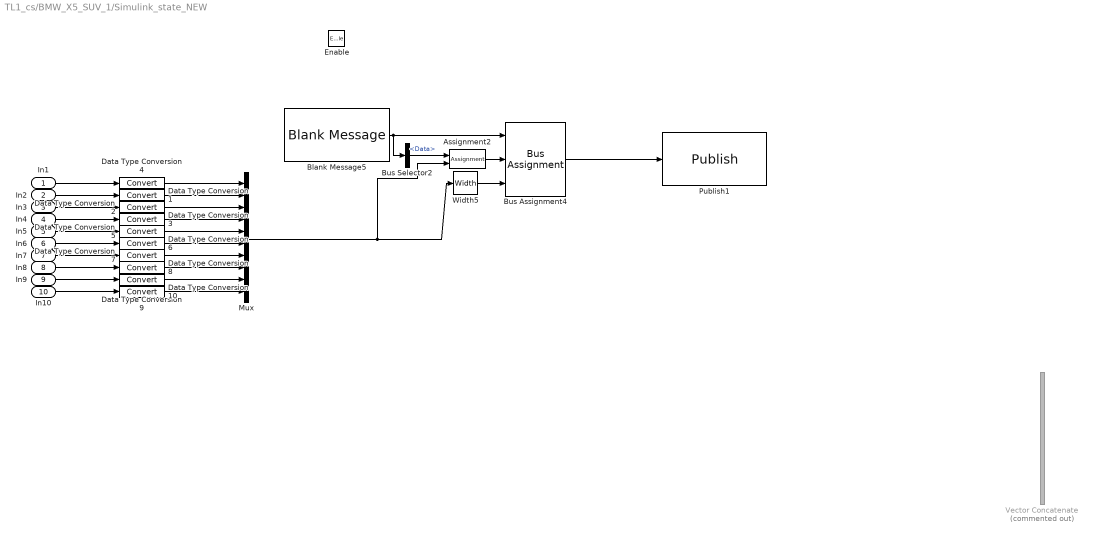
== system TL1_cs/BMW_X5_SUV_1/Simulink_state_NEW ==
  In1 : Inport
  In2 : Inport  Port=2
  In3 : Inport  Port=3
  In4 : Inport  Port=4
  In5 : Inport  Port=5
  In6 : Inport  Port=6
  In7 : Inport  Port=7
  In8 : Inport  Port=8
  In9 : Inport  Port=9
  In10 : Inport  Port=10
  Enable : EnablePort
  Assignment2 : Assignment  OutputInitialize=Specify size for each dimension in table  DiagnosticForDimensions=Warning  IndexOptions=Starting index (dialog)  Indices=1  OutputSizes=1000
  Blank Message5 : robotlib/Blank Message  messageClass=Message  entityType=std_msgs/Int32MultiArray  messageType=std_msgs/Int32MultiArray  SampleTime=inf
      settings: SourceProductBaseCode=RO
  Bus Assignment4 : BusAssignment  AssignedSignals=Data,Data_SL_Info.CurrentLength
  Bus Selector2 : BusSelector  OutputSignals=Data
  Data Type Conversion{1..10} (10 alike) : DataTypeConversion
  Mux : Mux  Inputs=10
  Publish1 : robotlib/Publish  topicSource=Specify your own  topic=/Simulink_state  messageType=std_msgs/Int32MultiArray  messageQueueLength=1
      settings: SourceProductBaseCode=RO
  Vector Concatenate : Concatenate  Commented=on  NumInputs=10
  Width5 : Width  DataType=uint32
  wires:
  In1/1 -> Data Type Conversion4/1
  Data Type Conversion4/1 -> Mux/1
  Bus Assignment4/1 -> Publish1/1
  Mux/1 -> Assignment2/2, Width5/1
  Width5/1 -> Bus Assignment4/3
  Data Type Conversion1/1 -> Mux/2
  Data Type Conversion2/1 -> Mux/3
  Data Type Conversion3/1 -> Mux/4
  Data Type Conversion5/1 -> Mux/5
  Data Type Conversion6/1 -> Mux/6
  Data Type Conversion7/1 -> Mux/7
  Data Type Conversion8/1 -> Mux/8
  Data Type Conversion9/1 -> Mux/9
  Data Type Conversion10/1 -> Mux/10
  In2/1 -> Data Type Conversion1/1
  In3/1 -> Data Type Conversion2/1
  In4/1 -> Data Type Conversion3/1
  In5/1 -> Data Type Conversion5/1
  In6/1 -> Data Type Conversion6/1
  In8/1 -> Data Type Conversion8/1
  In9/1 -> Data Type Conversion9/1
  In10/1 -> Data Type Conversion10/1
  In7/1 -> Data Type Conversion7/1
  Bus Selector2/1 -> Assignment2/1  "<Data>"
  Blank Message5/1 -> Bus Selector2/1, Bus Assignment4/1
  Assignment2/1 -> Bus Assignment4/2

== system TL1_cs/BMW_X5_SUV_1/Subsystem ==
  In1 : Inport
  In2 : Inport  Port=2
  In3 : Inport  Port=3
  In4 : Inport  Port=4
  In5 : Inport  Port=5
  Matrix Concatenate5 : Concatenate  NumInputs=4  Mode=Multidimensional array  ConcatenateDimension=2
  Reshape{1..4} (4 alike) : Reshape
  Rotate over Z : Subsystem
  Spherical to cartesian : Subsystem
  Out1 : Outport
  wires:
  In5/1 -> Reshape3/1
  Reshape4/1 -> Spherical to cartesian/1(In1)
  In1/1 -> Rotate over Z/1(In1)
  Reshape1/1 -> Spherical to cartesian/2(In2)
  Spherical to cartesian/1(Out1) -> Rotate over Z/2(In2)
  Reshape2/1 -> Spherical to cartesian/3(In3)
  Spherical to cartesian/2(Out2) -> Rotate over Z/3(In3)
  In3/1 -> Reshape1/1
  Rotate over Z/2(Out2) -> Matrix Concatenate5/2
  Spherical to cartesian/3(Out3) -> Matrix Concatenate5/3
  Reshape3/1 -> Matrix Concatenate5/4
  Rotate over Z/1(Out1) -> Matrix Concatenate5/1
  Matrix Concatenate5/1 -> Out1/1
  In2/1 -> Reshape4/1
  In4/1 -> Reshape2/1

== system TL1_cs/BMW_X5_SUV_1/Subsystem1 ==
  In1 : Inport
  In2 : Inport  Port=2
  In3 : Inport  Port=3
  In4 : Inport  Port=4
  In5 : Inport  Port=5
  Matrix Concatenate5 : Concatenate  NumInputs=4  Mode=Multidimensional array  ConcatenateDimension=2
  Reshape{1..4} (4 alike) : Reshape
  Rotate over Z : Subsystem
  Spherical to cartesian : Subsystem
  Out1 : Outport
  wires:
  In5/1 -> Reshape3/1
  Reshape4/1 -> Spherical to cartesian/1(In1)
  In1/1 -> Rotate over Z/1(In1)
  Reshape1/1 -> Spherical to cartesian/2(In2)
  Spherical to cartesian/1(Out1) -> Rotate over Z/2(In2)
  Reshape2/1 -> Spherical to cartesian/3(In3)
  Spherical to cartesian/2(Out2) -> Rotate over Z/3(In3)
  In3/1 -> Reshape1/1
  Rotate over Z/2(Out2) -> Matrix Concatenate5/2
  Spherical to cartesian/3(Out3) -> Matrix Concatenate5/3
  Reshape3/1 -> Matrix Concatenate5/4
  Rotate over Z/1(Out1) -> Matrix Concatenate5/1
  Matrix Concatenate5/1 -> Out1/1
  In2/1 -> Reshape4/1
  In4/1 -> Reshape2/1
